simulink model "ImpedanceScanAndRecord"  (R2020a)
settings: Solver=FixedStepDiscrete  StartTime=0.0  StopTime=30  FixedStep=Ts  RelTol=1e-3
InitFcn:
  | Ts = 50e-6
undefined symbols (not defined in the file or in its folder): DiscIntNeverNeededParam
libraries: dspsigops x10, powerlib x8
settings Model: SimulationMode=accelerator  Creator=anony  LastModifiedBy=anony

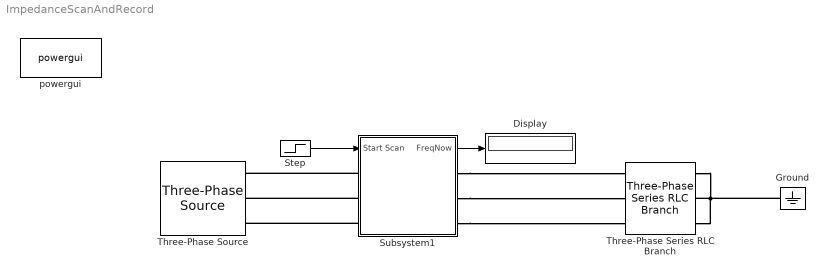
== system ImpedanceScanAndRecord ==
  Display : Display
  Ground : powerlib/Elements/Ground  LConnTagsString=a
  Step : Step  SampleTime=Ts
  Subsystem1 : Subsystem  mask{t_disturbance=2, t_wait4stable=1, t_record=1, amp_disturbance=37e3 * 0.02, vector_disturbance=[1:10], t_Ts=Ts}
      mask prompts: t_disturbance "扰动时间 (s)"; t_wait4stable "稳定时间 (s)"; t_record "录波时长 (s)"; amp_disturbance "扰动幅度 eg. 37e3*0.02"; vector_disturbance "扰动频率 (Hz) eg. [1:250], 1~250Hz"; t_Ts "Sample Time"
      mask help:
      | Impedance scan module
      | It generates voltage disturbance and reocord it as .mat file and variable.
      | This module DO NOT yield Impedance-Frequency characteristic directly, another .m file would be needed for postprocess.
      |
      | Yamin, created on 2020/05/03
  Three-Phase Series RLC Branch : powerlib/Elements/Three-Phase Series RLC Branch  LConnTagsString=A|B|C  RConnTagsString=A|B|C  BranchType=RL  Resistance=1  Inductance=1e-2  Capacitance=1e-6  Measurements=None
  Three-Phase Source : powerlib/Electrical Sources/Three-Phase Source  InternalConnection=Yg  VoltagePhases=off  Voltage=37e3  PhaseAngle=0  Voltage_phases=[25e3 25e3 25e3]/sqrt(3)  PhaseAngles_phases=[0 -120 +120]  Frequency=50  NonIdealSource=off  SpecifyImpedance=off  Resistance=0.8929  Inductance=16.58e-3  ShortCircuitLevel=100e6  BaseVoltage=25e3  XRratio=7  BusType=swing  Pref=10e3  Qref=0  Prefabc=[10e3, 10e3, 10e3]  Qrefabc=[0, 0, 0]  Qmin=-inf  Qmax=inf
  powergui : powerlib/powergui  Priority=1  SimulationMode=Discrete  SampleTime=Ts  frequency=60  Iterations=50  frequencyindice=0  Pbase=100e6  ErrMax=1e-4  UnitsV=kV  UnitsW=MW  buscounter=0  FunctionMessages=off  echomessages=off  EnableUseOfTLC=off  CurrentSourceSwitches=off  DisableSnubberDevices=off  DisableRonSwitches=off  DisableVfSwitches=off  DisplayEquations=off  AutomaticDiscreteSolvers=off  SolverType=Tustin/Backward Euler (TBE)  Interpol=off  ExternalGateDelay=off  methode=off  Ts=100  x0status=blocks  SPID=on  SwTol=0  HookPort=off  NonlinearTolerance=1e-4  nMaxIteration=100  ContinueOnMaxIteration=off  RestoreLinks=warning  ResistiveCurrentMeasurement=off  Frange=[0:2:500]  Ylog=off  Xlog=on  ShowGrid=off  save=off  variable=ZData  structure=0  ZoomFFT=off  StartTime=0.0  cycles=1  DisplayStyle=1  fundamental=60  FreqAxis=off  MaxFrequency=1000  frequencyindicesteady=1  RmsSteady=1  display=off
  wires:
  Step/1 -> Subsystem1/1(Start Scan)
  Subsystem1/1(FreqNow) -> Display/1
  connections:
  Ground/LConn1 -- Three-Phase Series RLC Branch/RConn3 -- Three-Phase Series RLC Branch/RConn1 -- Three-Phase Series RLC Branch/RConn2
  Subsystem1/RConn2 -- Three-Phase Series RLC Branch/LConn2
  Subsystem1/RConn1 -- Three-Phase Series RLC Branch/LConn1
  Subsystem1/RConn3 -- Three-Phase Series RLC Branch/LConn3
  Subsystem1/LConn2 -- Three-Phase Source/RConn2
  Subsystem1/LConn1 -- Three-Phase Source/RConn1
  Subsystem1/LConn3 -- Three-Phase Source/RConn3

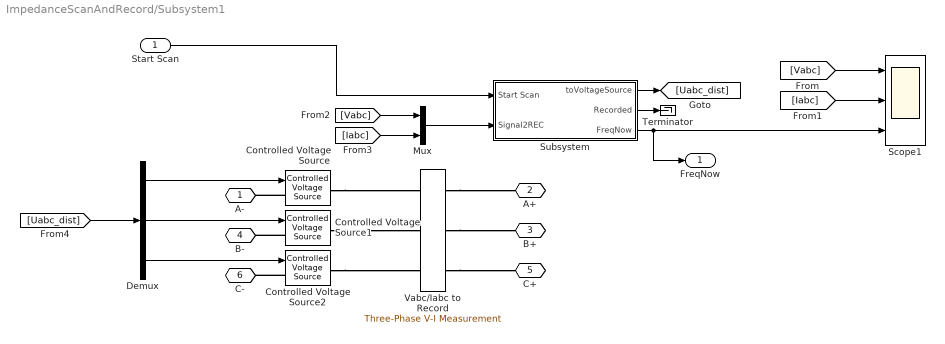
== system ImpedanceScanAndRecord/Subsystem1 ==
  Start Scan : Inport
  Controlled Voltage Source : powerlib/Electrical Sources/Controlled Voltage Source  Initialize=on  Source_Type=AC  Amplitude=0  Phase=0  Frequency=0  Measurements=None
  Controlled Voltage Source1 : powerlib/Electrical Sources/Controlled Voltage Source  Initialize=on  Source_Type=AC  Amplitude=0  Phase=0  Frequency=0  Measurements=None
  Controlled Voltage Source2 : powerlib/Electrical Sources/Controlled Voltage Source  Initialize=on  Source_Type=AC  Amplitude=0  Phase=0  Frequency=0  Measurements=None
  Demux : Demux  Outputs=3
  Mux : Mux  Inputs=2
  Scope1 : Scope  NumInputPorts=3
  Subsystem : Subsystem  mask{t_disturbance=t_disturbance, t_wait4stable=t_wait4stable, t_record=t_record, amp_disturbance=amp_disturbance, vector_freq=vector_disturbance, t_Ts=t_Ts}
      mask prompts: t_disturbance "扰动时长 (t)"; t_wait4stable "稳定时长 (t)"; t_record "录波时长 (t)"; amp_disturbance "扰动幅度 eg. 37e3 * 0.02 (37kV的2%)"; vector_freq "扰动频率 (Hz) eg. [1:250]"; t_Ts "Sample Time"
  Terminator : Terminator
  Vabc/Iabc to Record : powerlib/Measurements/Three-Phase V-I Measurement  VoltageMeasurement=phase-to-ground  SetLabelV=on  LabelV=Vabc  Vpu=off  VpuLL=off  CurrentMeasurement=yes  SetLabelI=on  LabelI=Iabc  Ipu=off  Pbase=100e6  Vbase=500e3  OutputType=Complex  PhasorSimulation=off  PSBequivalent=0
  A- : PMIOPort  Side=Left
  A+ : PMIOPort  Port=2  Side=Right
  B+ : PMIOPort  Port=3  Side=Right
  B- : PMIOPort  Port=4  Side=Left
  C+ : PMIOPort  Port=5  Side=Right
  C- : PMIOPort  Port=6  Side=Left
  FreqNow : Outport
  wires:
  Mux/1 -> Subsystem/2(Signal2REC)
  [Vabc] -> Mux/1
  Subsystem/2(Recorded) -> Terminator/1
  Demux/2 -> Controlled Voltage Source1/1
  [Iabc] -> Scope1/2
  Subsystem/3(FreqNow) -> FreqNow/1, Scope1/3
  [Vabc] -> Scope1/1
  [Iabc] -> Mux/2
  Subsystem/1(toVoltageSource) -> [Uabc_dist]
  Start Scan/1 -> Subsystem/1(Start Scan)
  Demux/1 -> Controlled Voltage Source/1
  Demux/3 -> Controlled Voltage Source2/1
  [Uabc_dist] -> Demux/1
  connections:
  Controlled Voltage Source/RConn1 -- Vabc/Iabc to Record/LConn1
  Controlled Voltage Source1/RConn1 -- Vabc/Iabc to Record/LConn2
  Vabc/Iabc to Record/RConn2 -- B+/RConn1
  Controlled Voltage Source2/RConn1 -- Vabc/Iabc to Record/LConn3
  Controlled Voltage Source2/LConn1 -- C-/RConn1
  Vabc/Iabc to Record/RConn3 -- C+/RConn1
  Vabc/Iabc to Record/RConn1 -- A+/RConn1
  Controlled Voltage Source/LConn1 -- A-/RConn1
  Controlled Voltage Source1/LConn1 -- B-/RConn1

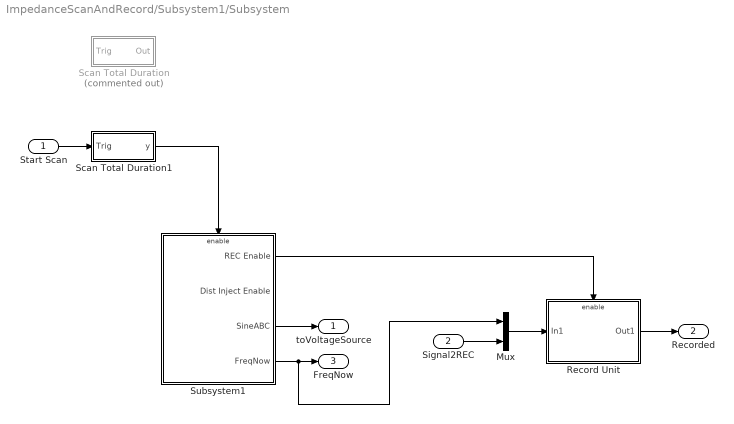
== system ImpedanceScanAndRecord/Subsystem1/Subsystem ==
  Start Scan : Inport
  Signal2REC : Inport  Port=2
  Mux : Mux  Inputs=2
  Record Unit : Subsystem
  Scan Total Duration : Subsystem  Commented=on  mask{time_delay=0, duration=(t_disturbance + t_wait4stable)*length(vector_freq)}
      mask prompts: time_delay "Time Delay (s)"; duration "Duration (s)"
      mask help:
      | Generating specific time duration pulse after a given time delay, rising-edge triggered.
      | Yamin, 2020/3/6
      mask Help: No help
      mask DialogControl DescTextVar Prompt: Generating specific time duration pulse after a given time delay, rising-edge triggered.
  Scan Total Duration1 : Subsystem  mask{time_delay=0, duration=(t_disturbance + t_wait4stable)*length(vector_freq)}
      mask prompts: time_delay "Time Delay (s)"; duration "Duration (s)"
      mask help:
      | Generating specific time duration pulse after a given time delay, rising-edge triggered.
      | Yamin, 2020/3/6
      mask Help: No help
      mask DialogControl DescTextVar Prompt: Generating specific time duration pulse after a given time delay, rising-edge triggered.
  Subsystem1 : Subsystem
  toVoltageSource : Outport
  Recorded : Outport  Port=2
  FreqNow : Outport  Port=3
  wires:
  Scan Total Duration1/1(y) -> Subsystem1/Enable
  Subsystem1/1(REC Enable) -> Record Unit/Enable
  Subsystem1/3(SineABC) -> toVoltageSource/1
  Record Unit/1(Out1) -> Recorded/1
  Start Scan/1 -> Scan Total Duration1/1(Trig)
  Subsystem1/4(FreqNow) -> Mux/1, FreqNow/1
  Mux/1 -> Record Unit/1(In1)
  Signal2REC/1 -> Mux/2

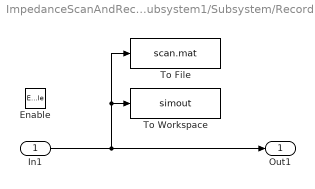
== system ImpedanceScanAndRecord/Subsystem1/Subsystem/Record Unit ==
  In1 : Inport
  Enable : EnablePort
  To File : ToFile  Filename=scan.mat  MatrixName=scan
  To Workspace : ToWorkspace  VariableName=simout  SampleTime=-1
  Out1 : Outport
  wires:
  In1/1 -> Out1/1, To File/1, To Workspace/1

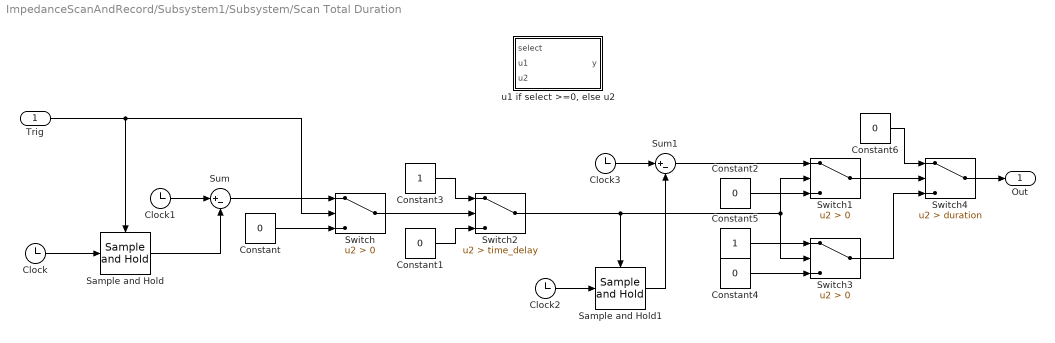
== system ImpedanceScanAndRecord/Subsystem1/Subsystem/Scan Total Duration ==
  Trig : Inport
  Clock{,1..3} (4 alike) : Clock
  Constant{,1..2,4,6} (5 alike) : Constant  Value=0
  Constant3 : Constant
  Constant5 : Constant
  Sample and Hold : dspsigops/Sample and Hold  trig=Rising edge  initCond=0  latchinput=off
  Sample and Hold1 : dspsigops/Sample and Hold  trig=Rising edge  initCond=0  latchinput=off
  Sum : Sum  Inputs=|+-
  Sum1 : Sum  Inputs=|+-
  Switch : Switch  Criteria=u2 > Threshold
  Switch1 : Switch  Criteria=u2 > Threshold
  Switch2 : Switch  Criteria=u2 > Threshold  Threshold=time_delay
  Switch3 : Switch  Criteria=u2 > Threshold
  Switch4 : Switch  Criteria=u2 > Threshold  Threshold=duration
  "u1 if select >=0, else u2" : MATLAB Function  TreatAsAtomicUnit=on  SystemSampleTime=Ts
  Out : Outport
  wires:
  Switch4/1 -> Out/1
  Switch3/1 -> Switch4/3
  Constant6/1 -> Switch4/1
  Switch1/1 -> Switch4/2
  Sum1/1 -> Switch1/1
  Switch2/1 -> Sample and Hold1/Trigger, Switch3/2, Switch1/2
  Constant5/1 -> Switch3/1
  Constant4/1 -> Switch3/3
  Constant2/1 -> Switch1/3
  Sample and Hold1/1 -> Sum1/2
  Clock3/1 -> Sum1/1
  Clock2/1 -> Sample and Hold1/1
  Clock/1 -> Sample and Hold/1
  Clock1/1 -> Sum/1
  Sample and Hold/1 -> Sum/2
  Constant/1 -> Switch/3
  Sum/1 -> Switch/1
  Trig/1 -> Sample and Hold/Trigger, Switch/2
  Switch/1 -> Switch2/2
  Constant3/1 -> Switch2/1
  Constant1/1 -> Switch2/3

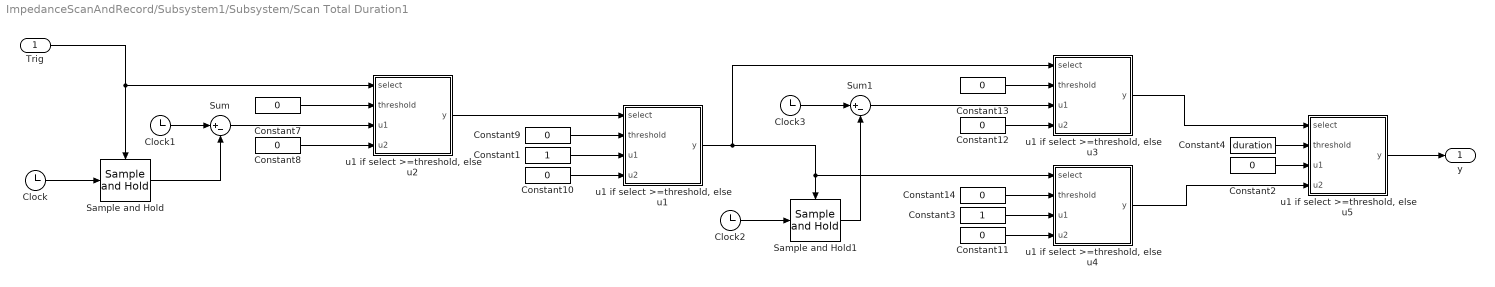
== system ImpedanceScanAndRecord/Subsystem1/Subsystem/Scan Total Duration1 ==
  Trig : Inport
  Clock{,1..3} (4 alike) : Clock
  Constant1 : Constant
  Constant{2,7..14} (9 alike) : Constant  Value=0
  Constant3 : Constant
  Constant4 : Constant  Value=duration
  Sample and Hold : dspsigops/Sample and Hold  trig=Rising edge  initCond=0  latchinput=off
  Sample and Hold1 : dspsigops/Sample and Hold  trig=Rising edge  initCond=0  latchinput=off
  Sum : Sum  Inputs=|+-
  Sum1 : Sum  Inputs=|+-
  "u1 if select >=threshold, else u1" : MATLAB Function  TreatAsAtomicUnit=on  SystemSampleTime=Ts
  "u1 if select >=threshold, else u2" : MATLAB Function  TreatAsAtomicUnit=on  SystemSampleTime=Ts
  "u1 if select >=threshold, else u3" : MATLAB Function  TreatAsAtomicUnit=on  SystemSampleTime=Ts
  "u1 if select >=threshold, else u4" : MATLAB Function  TreatAsAtomicUnit=on  SystemSampleTime=Ts
  "u1 if select >=threshold, else u5" : MATLAB Function  TreatAsAtomicUnit=on  SystemSampleTime=Ts
  y : Outport
  wires:
  Trig/1 -> Sample and Hold/Trigger, "u1 if select >=threshold, else u2"/1(select)
  Sum/1 -> "u1 if select >=threshold, else u2"/3(u1)
  Constant8/1 -> "u1 if select >=threshold, else u2"/4(u2)
  Sample and Hold/1 -> Sum/2
  Clock1/1 -> Sum/1
  Clock/1 -> Sample and Hold/1
  Clock2/1 -> Sample and Hold1/1
  Clock3/1 -> Sum1/1
  Sample and Hold1/1 -> Sum1/2
  "u1 if select >=threshold, else u1"/1(y) -> "u1 if select >=threshold, else u4"/1(select), Sample and Hold1/Trigger, "u1 if select >=threshold, else u3"/1(select)
  "u1 if select >=threshold, else u5"/1(y) -> y/1
  Constant7/1 -> "u1 if select >=threshold, else u2"/2(threshold)
  "u1 if select >=threshold, else u2"/1(y) -> "u1 if select >=threshold, else u1"/1(select)
  Constant9/1 -> "u1 if select >=threshold, else u1"/2(threshold)
  Constant10/1 -> "u1 if select >=threshold, else u1"/4(u2)
  Constant1/1 -> "u1 if select >=threshold, else u1"/3(u1)
  Constant3/1 -> "u1 if select >=threshold, else u4"/3(u1)
  Constant11/1 -> "u1 if select >=threshold, else u4"/4(u2)
  Constant12/1 -> "u1 if select >=threshold, else u3"/4(u2)
  Sum1/1 -> "u1 if select >=threshold, else u3"/3(u1)
  Constant13/1 -> "u1 if select >=threshold, else u3"/2(threshold)
  Constant14/1 -> "u1 if select >=threshold, else u4"/2(threshold)
  "u1 if select >=threshold, else u3"/1(y) -> "u1 if select >=threshold, else u5"/1(select)
  "u1 if select >=threshold, else u4"/1(y) -> "u1 if select >=threshold, else u5"/4(u2)
  Constant2/1 -> "u1 if select >=threshold, else u5"/3(u1)
  Constant4/1 -> "u1 if select >=threshold, else u5"/2(threshold)

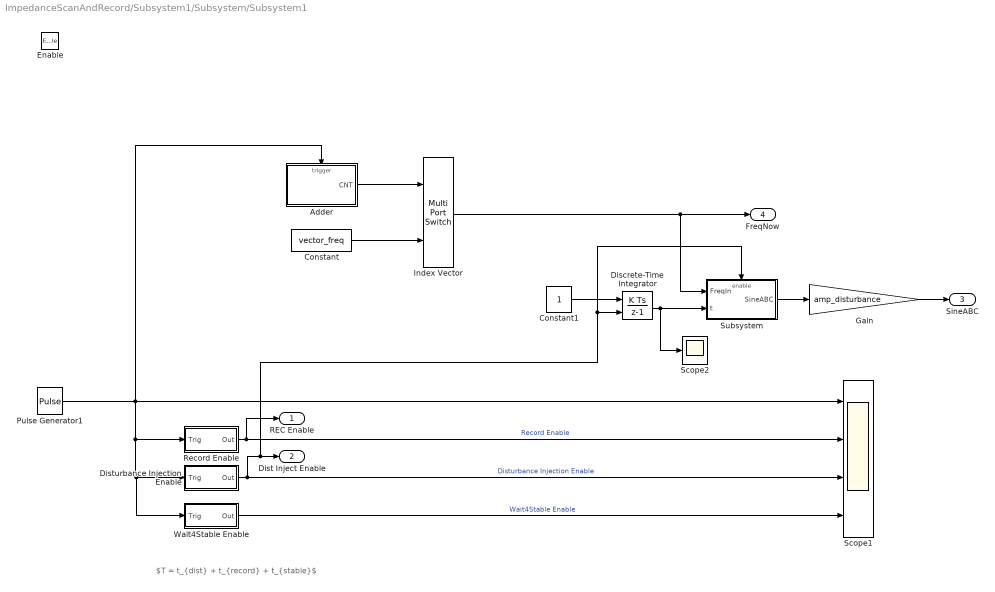
== system ImpedanceScanAndRecord/Subsystem1/Subsystem/Subsystem1 ==
  note: $T = t_{dist} + t_{record} + t_{stable}$
  Enable : EnablePort
  Adder : Subsystem
  Constant : Constant  Value=vector_freq
  Constant1 : Constant
  Discrete-Time Integrator : DiscreteIntegrator  gainval=1  ExternalReset=rising  SampleTime=t_Ts  ICPrevOutput=DiscIntNeverNeededParam  ICPrevScaledInput=DiscIntNeverNeededParam
  Disturbance Injection Enable : Subsystem  mask{time_delay=0, duration=t_disturbance}
      mask prompts: time_delay "Time Delay (s)"; duration "Duration (s)"
      mask help:
      | Generating specific time duration pulse after a given time delay, rising-edge triggered.
      | Yamin, 2020/3/6
      mask Help: No help
      mask DialogControl DescTextVar Prompt: Generating specific time duration pulse after a given time delay, rising-edge triggered.
  Gain : Gain  Gain=amp_disturbance
  Index Vector : MultiPortSwitch  DataPortOrder=Zero-based contiguous  Inputs=1  zeroidx=on
  Pulse Generator1 : DiscretePulseGenerator  PulseType=Time based  Period=t_disturbance + t_wait4stable  PulseWidth=99  PhaseDelay=t_Ts
  Record Enable : Subsystem  mask{time_delay=t_disturbance - t_record, duration=t_record}
      mask prompts: time_delay "Time Delay (s)"; duration "Duration (s)"
      mask help:
      | Generating specific time duration pulse after a given time delay, rising-edge triggered.
      | Yamin, 2020/3/6
      mask Help: No help
      mask DialogControl DescTextVar Prompt: Generating specific time duration pulse after a given time delay, rising-edge triggered.
  Scope1 : Scope  NumInputPorts=4
  Scope2 : Scope
  Subsystem : Subsystem
  Wait4Stable Enable : Subsystem  mask{time_delay=t_disturbance, duration=t_wait4stable}
      mask prompts: time_delay "Time Delay (s)"; duration "Duration (s)"
      mask help:
      | Generating specific time duration pulse after a given time delay, rising-edge triggered.
      | Yamin, 2020/3/6
      mask Help: No help
      mask DialogControl DescTextVar Prompt: Generating specific time duration pulse after a given time delay, rising-edge triggered.
  REC Enable : Outport
  Dist Inject Enable : Outport  Port=2
  SineABC : Outport  Port=3
  FreqNow : Outport  Port=4
  wires:
  Wait4Stable Enable/1(Out) -> Scope1/4  "Wait4Stable Enable"
  Disturbance Injection Enable/1(Out) -> Discrete-Time Integrator/2, Subsystem/Enable, Dist Inject Enable/1, Scope1/3  "Disturbance Injection Enable"
  Record Enable/1(Out) -> REC Enable/1, Scope1/2  "Record Enable"
  Pulse Generator1/1 -> Scope1/1, Adder/Trigger, Wait4Stable Enable/1(Trig), Disturbance Injection Enable/1(Trig), Record Enable/1(Trig)
  Adder/1(CNT) -> Index Vector/1
  Constant/1 -> Index Vector/2
  Constant1/1 -> Discrete-Time Integrator/1
  Discrete-Time Integrator/1 -> Scope2/1, Subsystem/2(t)
  Index Vector/1 -> FreqNow/1, Subsystem/1(FreqIn)
  Subsystem/1(SineABC) -> Gain/1
  Gain/1 -> SineABC/1

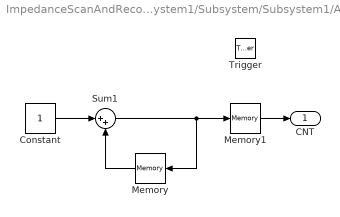
== system ImpedanceScanAndRecord/Subsystem1/Subsystem/Subsystem1/Adder ==
  Trigger : TriggerPort  VariantControl=Variant  PortDimensions=1
  Constant : Constant
  Memory : Memory  InheritSampleTime=on
  Memory1 : Memory  InheritSampleTime=on
  Sum1 : Sum  Inputs=|++
  CNT : Outport
  wires:
  Constant/1 -> Sum1/1
  Memory/1 -> Sum1/2
  Sum1/1 -> Memory1/1, Memory/1
  Memory1/1 -> CNT/1

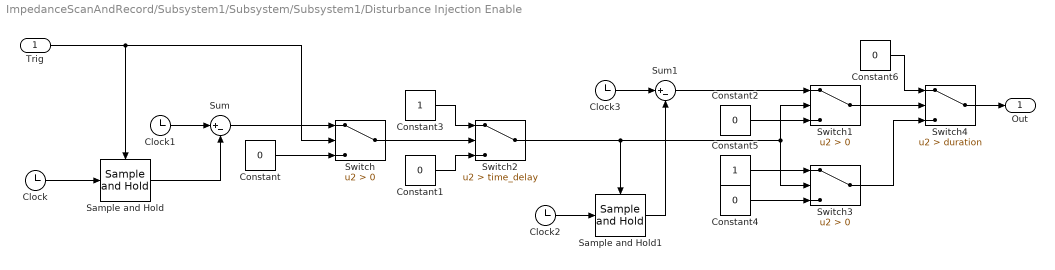
== system ImpedanceScanAndRecord/Subsystem1/Subsystem/Subsystem1/Disturbance Injection Enable ==
  Trig : Inport
  Clock{,1..3} (4 alike) : Clock
  Constant{,1..2,4,6} (5 alike) : Constant  Value=0
  Constant3 : Constant
  Constant5 : Constant
  Sample and Hold : dspsigops/Sample and Hold  trig=Rising edge  initCond=0  latchinput=off
  Sample and Hold1 : dspsigops/Sample and Hold  trig=Rising edge  initCond=0  latchinput=off
  Sum : Sum  Inputs=|+-
  Sum1 : Sum  Inputs=|+-
  Switch : Switch  Criteria=u2 > Threshold
  Switch1 : Switch  Criteria=u2 > Threshold
  Switch2 : Switch  Criteria=u2 > Threshold  Threshold=time_delay
  Switch3 : Switch  Criteria=u2 > Threshold
  Switch4 : Switch  Criteria=u2 > Threshold  Threshold=duration
  Out : Outport
  wires:
  Constant1/1 -> Switch2/3
  Constant3/1 -> Switch2/1
  Switch/1 -> Switch2/2
  Trig/1 -> Switch/2, Sample and Hold/Trigger
  Sum/1 -> Switch/1
  Constant/1 -> Switch/3
  Sample and Hold/1 -> Sum/2
  Clock1/1 -> Sum/1
  Clock/1 -> Sample and Hold/1
  Clock2/1 -> Sample and Hold1/1
  Clock3/1 -> Sum1/1
  Sample and Hold1/1 -> Sum1/2
  Constant2/1 -> Switch1/3
  Constant4/1 -> Switch3/3
  Constant5/1 -> Switch3/1
  Switch2/1 -> Switch1/2, Switch3/2, Sample and Hold1/Trigger
  Sum1/1 -> Switch1/1
  Switch1/1 -> Switch4/2
  Constant6/1 -> Switch4/1
  Switch3/1 -> Switch4/3
  Switch4/1 -> Out/1

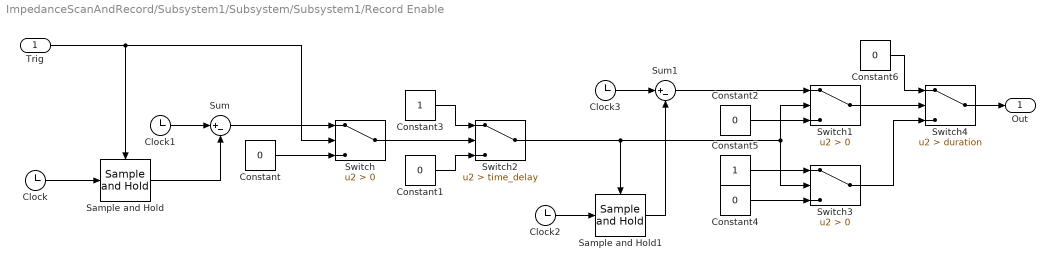
== system ImpedanceScanAndRecord/Subsystem1/Subsystem/Subsystem1/Record Enable ==
  Trig : Inport
  Clock{,1..3} (4 alike) : Clock
  Constant{,1..2,4,6} (5 alike) : Constant  Value=0
  Constant3 : Constant
  Constant5 : Constant
  Sample and Hold : dspsigops/Sample and Hold  trig=Rising edge  initCond=0  latchinput=off
  Sample and Hold1 : dspsigops/Sample and Hold  trig=Rising edge  initCond=0  latchinput=off
  Sum : Sum  Inputs=|+-
  Sum1 : Sum  Inputs=|+-
  Switch : Switch  Criteria=u2 > Threshold
  Switch1 : Switch  Criteria=u2 > Threshold
  Switch2 : Switch  Criteria=u2 > Threshold  Threshold=time_delay
  Switch3 : Switch  Criteria=u2 > Threshold
  Switch4 : Switch  Criteria=u2 > Threshold  Threshold=duration
  Out : Outport
  wires:
  Switch4/1 -> Out/1
  Switch3/1 -> Switch4/3
  Constant6/1 -> Switch4/1
  Switch1/1 -> Switch4/2
  Sum1/1 -> Switch1/1
  Switch2/1 -> Sample and Hold1/Trigger, Switch3/2, Switch1/2
  Constant5/1 -> Switch3/1
  Constant4/1 -> Switch3/3
  Constant2/1 -> Switch1/3
  Sample and Hold1/1 -> Sum1/2
  Clock3/1 -> Sum1/1
  Clock2/1 -> Sample and Hold1/1
  Clock/1 -> Sample and Hold/1
  Clock1/1 -> Sum/1
  Sample and Hold/1 -> Sum/2
  Constant/1 -> Switch/3
  Sum/1 -> Switch/1
  Trig/1 -> Sample and Hold/Trigger, Switch/2
  Switch/1 -> Switch2/2
  Constant3/1 -> Switch2/1
  Constant1/1 -> Switch2/3

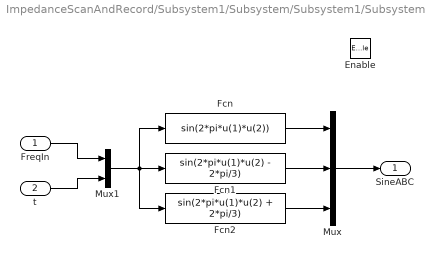
== system ImpedanceScanAndRecord/Subsystem1/Subsystem/Subsystem1/Subsystem ==
  FreqIn : Inport
  t : Inport  Port=2
  Enable : EnablePort
  Fcn : Fcn  Expr=sin(2*pi*u(1)*u(2))
  Fcn1 : Fcn  Expr=sin(2*pi*u(1)*u(2) - 2*pi/3)
  Fcn2 : Fcn  Expr=sin(2*pi*u(1)*u(2) + 2*pi/3)
  Mux : Mux  Inputs=3
  Mux1 : Mux  Inputs=2
  SineABC : Outport
  wires:
  Fcn1/1 -> Mux/2
  Fcn/1 -> Mux/1
  Fcn2/1 -> Mux/3
  Mux/1 -> SineABC/1
  Mux1/1 -> Fcn2/1, Fcn/1, Fcn1/1
  FreqIn/1 -> Mux1/1
  t/1 -> Mux1/2

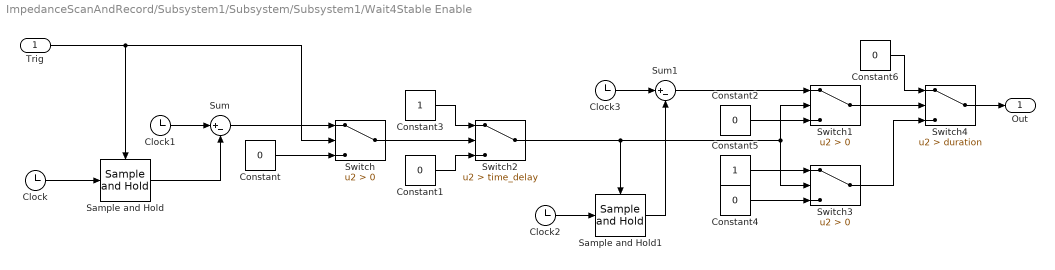
== system ImpedanceScanAndRecord/Subsystem1/Subsystem/Subsystem1/Wait4Stable Enable ==
  Trig : Inport
  Clock{,1..3} (4 alike) : Clock
  Constant{,1..2,4,6} (5 alike) : Constant  Value=0
  Constant3 : Constant
  Constant5 : Constant
  Sample and Hold : dspsigops/Sample and Hold  trig=Rising edge  initCond=0  latchinput=off
  Sample and Hold1 : dspsigops/Sample and Hold  trig=Rising edge  initCond=0  latchinput=off
  Sum : Sum  Inputs=|+-
  Sum1 : Sum  Inputs=|+-
  Switch : Switch  Criteria=u2 > Threshold
  Switch1 : Switch  Criteria=u2 > Threshold
  Switch2 : Switch  Criteria=u2 > Threshold  Threshold=time_delay
  Switch3 : Switch  Criteria=u2 > Threshold
  Switch4 : Switch  Criteria=u2 > Threshold  Threshold=duration
  Out : Outport
  wires:
  Switch4/1 -> Out/1
  Switch3/1 -> Switch4/3
  Constant6/1 -> Switch4/1
  Switch1/1 -> Switch4/2
  Sum1/1 -> Switch1/1
  Switch2/1 -> Sample and Hold1/Trigger, Switch3/2, Switch1/2
  Constant5/1 -> Switch3/1
  Constant4/1 -> Switch3/3
  Constant2/1 -> Switch1/3
  Sample and Hold1/1 -> Sum1/2
  Clock3/1 -> Sum1/1
  Clock2/1 -> Sample and Hold1/1
  Clock/1 -> Sample and Hold/1
  Clock1/1 -> Sum/1
  Sample and Hold/1 -> Sum/2
  Constant/1 -> Switch/3
  Sum/1 -> Switch/1
  Trig/1 -> Sample and Hold/Trigger, Switch/2
  Switch/1 -> Switch2/2
  Constant3/1 -> Switch2/1
  Constant1/1 -> Switch2/3

== matlab function ImpedanceScanAndRecord/Subsystem1/Subsystem/Scan Total Duration1/u1 if select >=threshold, else u2 ==
  data: select input; threshold input; u1 input; y output; u2 input
function y = fcn(select, threshold,u1, u2)
if select >= threshold
    y = u1;
else
    y = u2;
end

== matlab function ImpedanceScanAndRecord/Subsystem1/Subsystem/Scan Total Duration/u1 if select >=0, else u2 ==
  data: select input; u1 input; y output; u2 input
function y = fcn(select, u1, u2)
if select >= 1
    y = u1;
else
    y = u2;
end

== matlab function ImpedanceScanAndRecord/Subsystem1/Subsystem/Scan Total Duration1/u1 if select >=threshold, else u1 ==
  data: select input; threshold input; u1 input; y output; u2 input
function y = fcn(select, threshold,u1, u2)
if select >= threshold
    y = u1;
else
    y = u2;
end

== matlab function ImpedanceScanAndRecord/Subsystem1/Subsystem/Scan Total Duration1/u1 if select >=threshold, else u3 ==
  data: select input; threshold input; u1 input; y output; u2 input
function y = fcn(select, threshold,u1, u2)
if select >= threshold
    y = u1;
else
    y = u2;
end

== matlab function ImpedanceScanAndRecord/Subsystem1/Subsystem/Scan Total Duration1/u1 if select >=threshold, else u4 ==
  data: select input; threshold input; u1 input; y output; u2 input
function y = fcn(select, threshold,u1, u2)
if select >= threshold
    y = u1;
else
    y = u2;
end

== matlab function ImpedanceScanAndRecord/Subsystem1/Subsystem/Scan Total Duration1/u1 if select >=threshold, else u5 ==
  data: select input; threshold input; u1 input; y output; u2 input
function y = fcn(select, threshold,u1, u2)
if select >= threshold
    y = u1;
else
    y = u2;
end
